simulink model "pitch_hastighet"  (R2014b)
settings: Solver=ode1  StartTime=0.0  StopTime=10  FixedStep=0.1  RelTol=1e-3
values from neighbouring files (symbols this model uses):
  delta = pi/16    (= 0.196349540849)    [pitch_main.m]
  J = 15    [pitch_main.m]
  k = 100    [eulers_metode_d.m]    (also in eulers_metode_og_ekakt.m; pitch_main.m; sim_system.m)
  k_2 = 5    [pitch_main.m]
  k_3 = 1    [pitch_main.m]
  k_4 = 1    [pitch_main.m]
  m = 200    [eulers_metode_d.m]    (also in eulers_metode_og_ekakt.m; pitch_main.m; sim_system.m)
  theta_0 = pi/8    (= 0.392699081699)    [pitch_main.m]
  theta_dot0 = 0    [pitch_main.m]
  v_0 = 0    [pitch_main.m]    (also in sim_system.m)
libraries: simulink x1
settings Model: Creator=rende_000  LastModifiedBy=rende_000

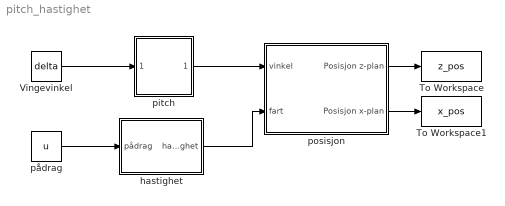
== system pitch_hastighet ==
  To Workspace : ToWorkspace  VariableName=z_pos  SaveFormat=Timeseries  SampleTime=-1
  To Workspace1 : ToWorkspace  VariableName=x_pos  SaveFormat=Timeseries  SampleTime=-1
  Vingevinkel : Constant  Value=delta
  hastighet : Subsystem
  pitch : Subsystem
  posisjon : Subsystem
  pådrag : Constant  Value=u
  wires:
  Vingevinkel/1 -> pitch/1(delta)
  pådrag/1 -> hastighet/1(pådrag)
  pitch/1(theta) -> posisjon/1(vinkel)
  hastighet/1(hastighet) -> posisjon/2(fart)
  posisjon/1(Posisjon z-plan) -> To Workspace/1
  posisjon/2(Posisjon x-plan) -> To Workspace1/1

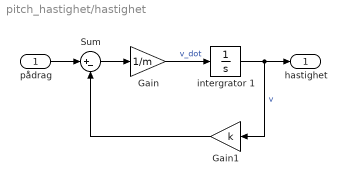
== system pitch_hastighet/hastighet ==
  pådrag : Inport
  Gain : Gain  Gain=1/m
  Gain1 : Gain  Gain=k
  Sum : Sum  Inputs=|+-
  intergrator 1 : Integrator  InitialCondition=v_0
  hastighet : Outport
  wires:
  intergrator 1/1 -> hastighet/1, Gain1/1  "v"
  Sum/1 -> Gain/1
  Gain/1 -> intergrator 1/1  "v_dot"
  pådrag/1 -> Sum/1
  Gain1/1 -> Sum/2

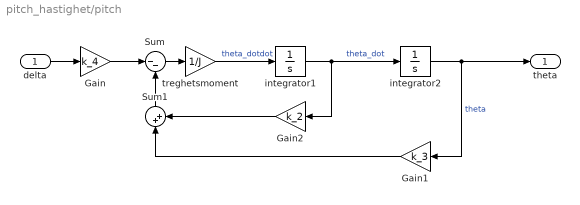
== system pitch_hastighet/pitch ==
  delta : Inport
  Gain : Gain  Gain=k_4
  Gain1 : Gain  Gain=k_3
  Gain2 : Gain  Gain=k_2
  Sum : Sum  Inputs=|--
  Sum1 : Sum  Inputs=|++
  integrator1 : Integrator  InitialCondition=theta_dot0
  integrator2 : Integrator  InitialCondition=theta_0
  treghetsmoment : Gain  Gain=1/J
  theta : Outport
  wires:
  Sum/1 -> treghetsmoment/1
  Sum1/1 -> Sum/2
  treghetsmoment/1 -> integrator1/1  "theta_dotdot"
  delta/1 -> Gain/1
  Gain/1 -> Sum/1
  Gain2/1 -> Sum1/2
  Gain1/1 -> Sum1/1
  integrator1/1 -> Gain2/1, integrator2/1  "theta_dot"
  integrator2/1 -> theta/1, Gain1/1  "theta"

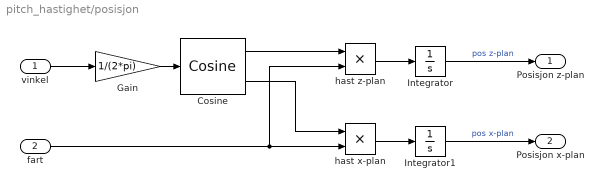
== system pitch_hastighet/posisjon ==
  vinkel : Inport
  fart : Inport  Port=2
  Cosine : simulink/Lookup Tables/Cosine  Formula=sin(2*pi*u) and cos(2*pi*u)  NumDataPoints=(2^5)+1  OutputWordLength=16  InternalRulePriority=Speed
  Gain : Gain  Gain=1/(2*pi)
  Integrator : Integrator
  Integrator1 : Integrator
  hast x-plan : Product
  hast z-plan : Product
  Posisjon z-plan : Outport
  Posisjon x-plan : Outport  Port=2
  wires:
  fart/1 -> hast z-plan/2, hast x-plan/2
  hast x-plan/1 -> Integrator1/1
  Cosine/2 -> hast x-plan/1
  Integrator1/1 -> Posisjon x-plan/1  "pos x-plan"
  hast z-plan/1 -> Integrator/1
  Gain/1 -> Cosine/1
  Cosine/1 -> hast z-plan/1
  Integrator/1 -> Posisjon z-plan/1  "pos z-plan"
  vinkel/1 -> Gain/1
